simulink subsystem "inner_subsys"  (R2025b)
settings: Solver=VariableStepAuto  StartTime=0.0  StopTime=10.0  RelTol=1e-3
undefined symbols (not defined in the file or in its folder): FL, WL
settings Model: Creator=Andrei  LastModifiedBy=Andrei

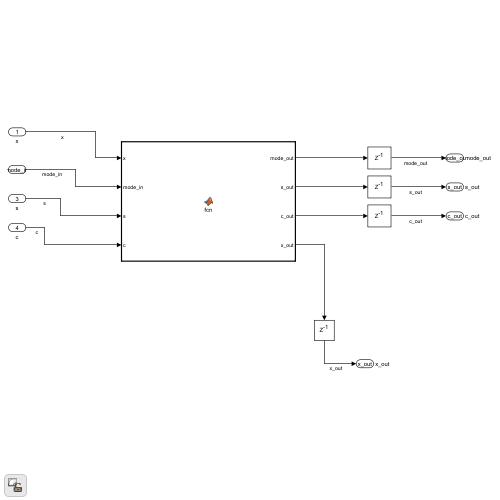
[thumbnail: Simulink's stored preview of the top-level diagram]
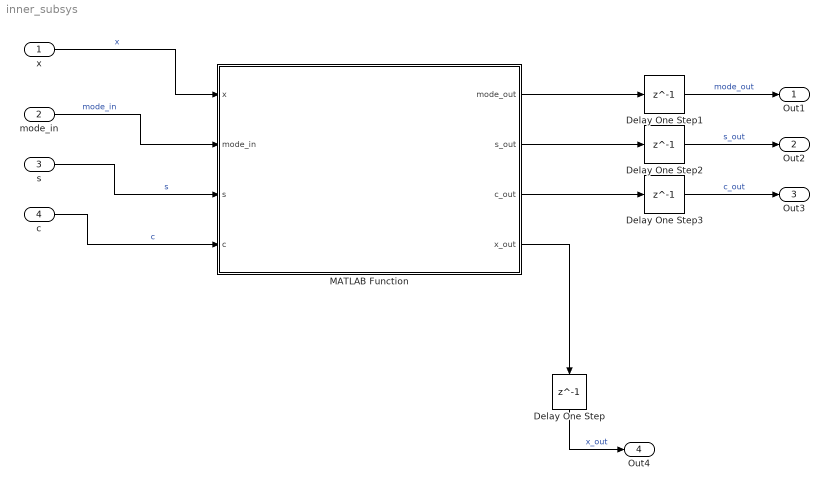
== system inner_subsys ==
  x : Inport
  mode_in : Inport  Port=2
  s : Inport  Port=3
  c : Inport  Port=4
  Delay One Step{,1..3} (4 alike) : Delay  DelayLength=1
  MATLAB Function : MATLAB Function  TreatAsAtomicUnit=on
  Out1 : Outport  SignalName=mode_out
  Out2 : Outport  Port=2  SignalName=s_out
  Out3 : Outport  Port=3  SignalName=c_out
  Out4 : Outport  Port=4  SignalName=x_out
  wires:
  Delay One Step/1 -> Out4/1  "x_out"
  MATLAB Function/2(s_out) -> Delay One Step2/1
  Delay One Step1/1 -> Out1/1  "mode_out"
  MATLAB Function/3(c_out) -> Delay One Step3/1
  MATLAB Function/1(mode_out) -> Delay One Step1/1
  x/1 -> MATLAB Function/1(x)  "x"
  c/1 -> MATLAB Function/4(c)  "c"
  MATLAB Function/4(x_out) -> Delay One Step/1
  Delay One Step2/1 -> Out2/1  "s_out"
  Delay One Step3/1 -> Out3/1  "c_out"
  s/1 -> MATLAB Function/3(s)  "s"
  mode_in/1 -> MATLAB Function/2(mode_in)  "mode_in"

== matlab function inner_subsys/MATLAB Function ==
  data: x input; mode_out output; mode_in input; s_out output; c_out output; x_out output; s input; c input; WL parameter; FL parameter
function [mode_out,s_out, c_out, x_out]    = fcn(x, mode_in, s,c, WL, FL)

T = numerictype(1, WL, FL);

x_fi = fi(x, T);
c_fi = fi(c, T);

persistent p_state;
if isempty(p_state)
    p_state = fi(0, 1, WL, FL);
end


s_out = s;
c_out = c;

if mode_in==1 % mode 1, conform articolului
    if s == 1
        x_out = p_state + c_fi*x_fi;
        p_state = x_fi;
    else
        x_out = x_fi + c_fi*p_state;
    end
else  
    x_out = x_fi + c_fi*p_state;
end

mode_out = mode_in;
